simulink model "questao01_pat"  (R2020a)
settings: Solver=VariableStepAuto  StartTime=0.0  StopTime=240  RelTol=1e-3
values from neighbouring files (symbols this model uses):
  A = [1 2 0;-1 -1 -1;0 2 -1]    [lqr_estudos.m]    (also in questao2_pat.m = [1 2 0; -1 -1 -1; 0 2 -1])
  B = [0;0;2]    [lqr_estudos.m]    (also in questao2_pat.m)
  C = [0 1 0;0 0 1]    [lqr_estudos.m]    (also in questao2_pat.m = [0 1 0; 0 0 1])
  K = place(A,B,poles)    [estudos_versao_laurinda.m]    (also in lqr_estudos.m = lqr(A,B,Q,R); questao1_pat.m = Ka(1:3); questao1_well.m = Ka(1:3); questao2_pat.m = place(A,B,newpoles))
  Kz = 1    [estudos_versao_laurinda.m]    (also in questao1_pat.m = Ka(4); questao1_well.m = Ka(4))
settings Model: Creator=wwagner  LastModifiedBy=patricia

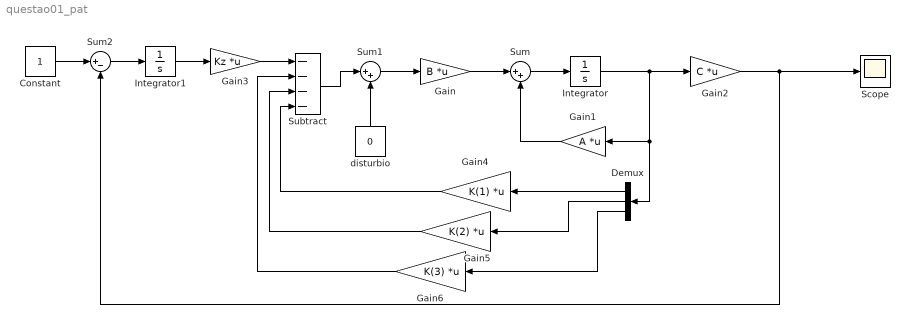
== system questao01_pat ==
  Constant : Constant
  Demux : Demux  Outputs=3
  Gain : Gain  Gain=B  Multiplication=Matrix(K*u)
  Gain1 : Gain  Gain=A  Multiplication=Matrix(K*u)
  Gain2 : Gain  Gain=C  Multiplication=Matrix(K*u)
  Gain3 : Gain  Gain=Kz  Multiplication=Matrix(K*u)
  Gain4 : Gain  Gain=K(1)  Multiplication=Matrix(K*u)
  Gain5 : Gain  Gain=K(2)  Multiplication=Matrix(K*u)
  Gain6 : Gain  Gain=K(3)  Multiplication=Matrix(K*u)
  Integrator : Integrator
  Integrator1 : Integrator
  Scope : Scope
  Subtract : Sum  Inputs=----
  Sum : Sum  Inputs=|++
  Sum1 : Sum  Inputs=|++
  Sum2 : Sum  Inputs=|+-
  disturbio : Constant  Value=0
  wires:
  Integrator/1 -> Demux/1, Gain1/1, Gain2/1
  Gain/1 -> Sum/1
  Gain1/1 -> Sum/2
  Sum/1 -> Integrator/1
  Gain2/1 -> Sum2/2, Scope/1
  Sum1/1 -> Gain/1
  Sum2/1 -> Integrator1/1
  Constant/1 -> Sum2/1
  Integrator1/1 -> Gain3/1
  Gain3/1 -> Subtract/1
  Subtract/1 -> Sum1/1
  disturbio/1 -> Sum1/2
  Gain4/1 -> Subtract/4
  Gain5/1 -> Subtract/3
  Gain6/1 -> Subtract/2
  Demux/1 -> Gain4/1
  Demux/2 -> Gain5/1
  Demux/3 -> Gain6/1
